simulink model "kalman_filter"  (R2016b)
settings: Solver=FixedStepDiscrete  StartTime=0.0  StopTime=10.0  FixedStep=0.1  RelTol=1e-3
undefined symbols (not defined in the file): InitialHeight, InitialHeightError, InitialHeightStd, InitialVelocity, InitialVelocityError, InitialVelocityStd, ObservationNoise, ProcessNoise, SpeedOfLight
settings Model: Creator=csax  LastModifiedBy=csax
settings OptimizationCC: DefaultParameterBehavior=Inlined
settings DebuggingCC: ParameterTunabilityLossMsg=error
settings HardwareCC: ProdBitPerPointer=32  ProdBitPerSizeT=32  ProdBitPerPtrDiffT=32  ProdLargestAtomicFloat=None  ProdWordSize=32  ProdHWDeviceType=Custom Processor->Custom
settings RTWCC: SystemTargetFile=trace32_target_ert.tlc  MakeCommand=trace32_target_make  TemplateMakefile=trace32_arm_tmf.tmf  Description=TRACE32 Target  GenerateReport=on  IncludeHyperlinkInReport=on  LaunchReport=on  GenerateTraceInfo=on  GenerateTraceReport=on  GenerateTraceReportSl=on  GenerateTraceReportSf=on  GenerateTraceReportEml=on
settings CodeAppCC: ForceParamTrailComments=on  IgnoreCustomStorageClasses=off  OperatorAnnotations=on  SimulinkDataObjDesc=on  SFDataObjDesc=on  MATLABFcnDesc=on  InsertBlockDesc=on  MATLABSourceComments=on
settings STFCustomTargetCC: TargetLangStandard=C99 (ISO)  CombineOutputUpdateFcns=on  ERTCustomFileBanners=on  SupportContinuousTime=off  SupportNonInlinedSFcns=off  RemoveResetFunc=on  MATLABClassNameForMDSCustomization=Simulink.SoftwareTarget.ERTCustomization  GRTInterface=off  SystemTargetFile=trace32_target_ert.tlc
settings ERTTargetCC: TargetLangStandard=C99 (ISO)  ParMdlRefBuildCompliant=off  CompOptLevelCompliant=off  ConcurrentExecutionCompliant=off  ERTFirstTimeCompliant=off  ModelStepFunctionPrototypeControlCompliant=off  CPPClassGenCompliant=off  UseToolchainInfoCompliant=off  InlinedParameterPlacement=NonHierarchical  ERTCustomFileTemplate=example_file_process.tlc

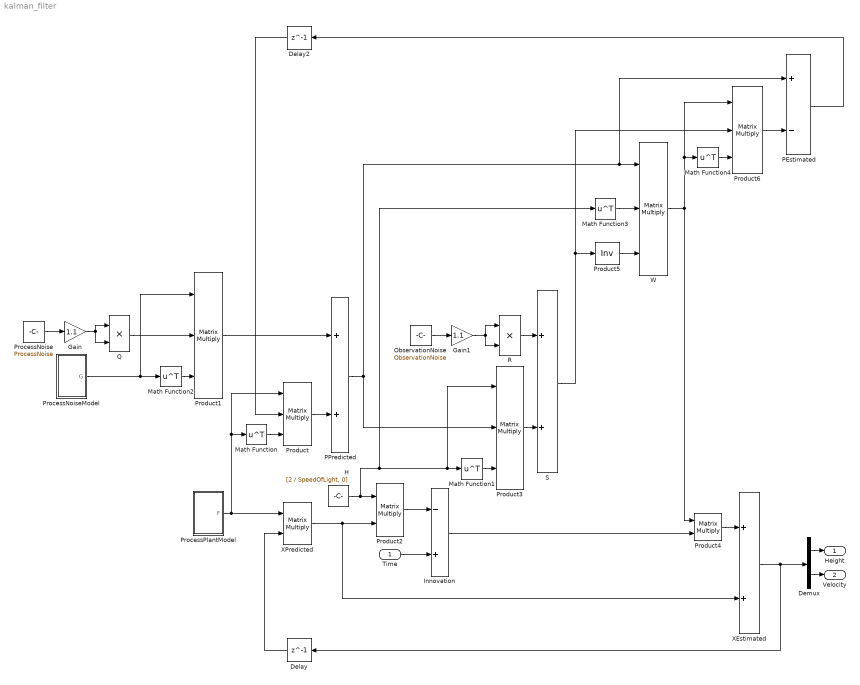
== system kalman_filter ==
  Time : Inport
  Delay : Delay  DelayLength=1  InitialCondition=[InitialHeight + InitialHeightError; InitialVelocity + InitialVelocityError]
  Delay2 : Delay  DelayLength=1  InitialCondition=[InitialHeightStd * InitialHeightStd, 0; 0, InitialVelocityStd * InitialVelocityStd]
  Demux : Demux  Outputs=2
  Gain : Gain  Gain=1.1
  Gain1 : Gain  Gain=1.1
  H : Constant  Value=[2 / SpeedOfLight, 0]  VectorParams1D=off  SampleTime=-1
  Innovation : Sum  Inputs=-+
  Math Function{,1..4} (5 alike) : Math  Operator=transpose  SaturateOnIntegerOverflow=on
  ObservationNoise : Constant  Value=ObservationNoise
  PEstimated : Sum  Inputs=+-
  PPredicted : Sum
  ProcessNoise : Constant  Value=ProcessNoise
  ProcessNoiseModel : Subsystem
  ProcessPlantModel : Subsystem
  Product{,1,3,6} (4 alike) : Product  Inputs=3  Multiplication=Matrix(*)
  Product2 : Product  Multiplication=Matrix(*)
  Product4 : Product  Multiplication=Matrix(*)
  Product5 : Product  Inputs=/  Multiplication=Matrix(*)
  Q : Product
  R : Product
  "S " : Sum
  W : Product  Inputs=3  Multiplication=Matrix(*)
  XEstimated : Sum
  XPredicted : Product  Multiplication=Matrix(*)
  Height : Outport
  Velocity : Outport  Port=2
  wires:
  ProcessNoise/1 -> Gain/1
  Gain/1 -> Q/2, Q/1
  ObservationNoise/1 -> Gain1/1
  Gain1/1 -> R/2, R/1
  ProcessPlantModel/1(F) -> Product/1, Math Function/1, XPredicted/1
  Delay/1 -> XPredicted/2
  Math Function/1 -> Product/3
  Delay2/1 -> Product/2
  Product/1 -> PPredicted/2
  ProcessNoiseModel/1(G) -> Math Function2/1, Product1/1
  Q/1 -> Product1/2
  Math Function2/1 -> Product1/3
  Product1/1 -> PPredicted/1
  H/1 -> Math Function3/1, Math Function1/1, Product3/1, Product2/1
  XPredicted/1 -> XEstimated/2, Product2/2
  Product2/1 -> Innovation/1
  Time/1 -> Innovation/2
  Math Function1/1 -> Product3/3
  PPredicted/1 -> PEstimated/1, W/1, Product3/2
  R/1 -> "S "/1
  Product3/1 -> "S "/2
  "S "/1 -> Product6/2, Product5/1
  Math Function3/1 -> W/2
  Product5/1 -> W/3
  W/1 -> Product4/1, Product6/1, Math Function4/1
  Innovation/1 -> Product4/2
  Product4/1 -> XEstimated/1
  XEstimated/1 -> Delay/1, Demux/1
  Math Function4/1 -> Product6/3
  PEstimated/1 -> Delay2/1
  Product6/1 -> PEstimated/2
  Demux/2 -> Velocity/1
  Demux/1 -> Height/1

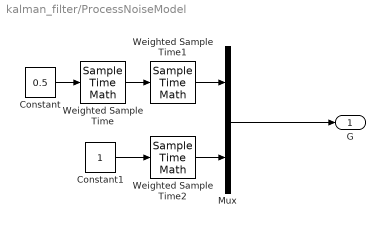
== system kalman_filter/ProcessNoiseModel ==
  Constant : Constant  Value=0.5
  Constant1 : Constant
  Mux : Mux  Inputs=2
  Weighted Sample Time : SampleTimeMath  TsampMathOp=*
  Weighted Sample Time1 : SampleTimeMath  TsampMathOp=*
  Weighted Sample Time2 : SampleTimeMath  TsampMathOp=Ts Only
  G : Outport
  wires:
  Weighted Sample Time/1 -> Weighted Sample Time1/1
  Constant/1 -> Weighted Sample Time/1
  Weighted Sample Time1/1 -> Mux/1
  Mux/1 -> G/1
  Weighted Sample Time2/1 -> Mux/2
  Constant1/1 -> Weighted Sample Time2/1

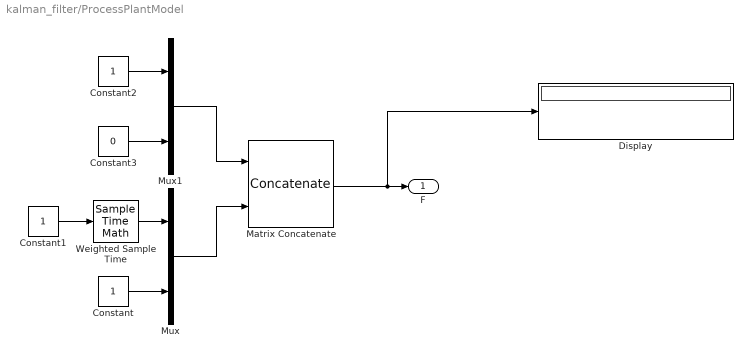
== system kalman_filter/ProcessPlantModel ==
  Constant : Constant
  Constant1 : Constant
  Constant2 : Constant
  Constant3 : Constant  Value=0
  Display : Display
  Matrix Concatenate : Concatenate  Mode=Multidimensional array  ConcatenateDimension=2
  Mux : Mux  Inputs=2
  Mux1 : Mux  Inputs=2
  Weighted Sample Time : SampleTimeMath  TsampMathOp=Ts Only
  F : Outport
  wires:
  Matrix Concatenate/1 -> Display/1, F/1
  Weighted Sample Time/1 -> Mux/1
  Constant/1 -> Mux/2
  Mux1/1 -> Matrix Concatenate/1
  Constant3/1 -> Mux1/2
  Mux/1 -> Matrix Concatenate/2
  Constant2/1 -> Mux1/1
  Constant1/1 -> Weighted Sample Time/1
